simulink model "Motor_pos_ref"  (R2020b)
settings: Solver=ode45  StartTime=0.0  StopTime=0.2  RelTol=1e-3
values from neighbouring files (symbols this model uses):
  b = 3.5077E-6    [DataDictionary.sldd]
  J = 3.2284E-6    [DataDictionary.sldd]
  Ke = 0.0274    [DataDictionary.sldd]
  Kt = 0.0274    [DataDictionary.sldd]
  L = 2.75E-6    [DataDictionary.sldd]
  R = 4.0    [DataDictionary.sldd]
settings Model: DataDictionary=DataDictionary.sldd  PacingRate=1000000  Creator=abhin  LastModifiedBy=abhin
settings DataIOCC: SaveOutput=off  SaveTime=off

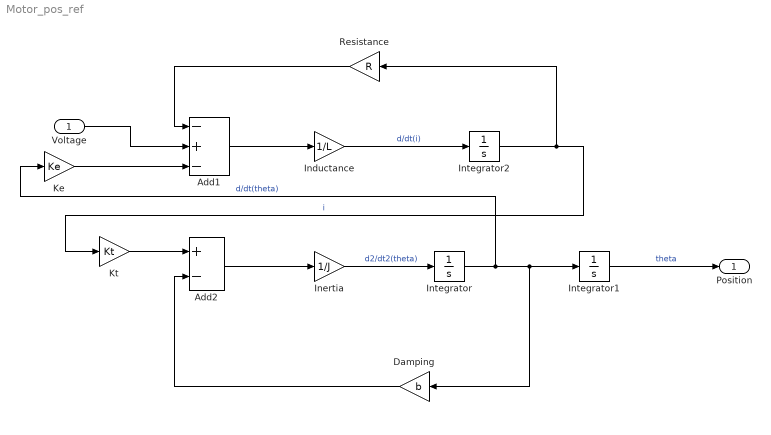
== system Motor_pos_ref ==
  Voltage : Inport  OutDataTypeStr=double  PortDimensions=1  SampleTime=0
  Add1 : Sum  Inputs=-+-
  Add2 : Sum  Inputs=+-
  Damping : Gain  Gain=b
  Inductance : Gain  Gain=1/L
  Inertia : Gain  Gain=1/J
  Integrator : Integrator
  Integrator1 : Integrator
  Integrator2 : Integrator
  Ke : Gain  Gain=Ke
  Kt : Gain  Gain=Kt
  Resistance : Gain  Gain=R
  Position : Outport  OutDataTypeStr=double  PortDimensions=1  SampleTime=0
  wires:
  Integrator1/1 -> Position/1  "theta"
  Inductance/1 -> Integrator2/1  "d/dt(i)"
  Integrator2/1 -> Kt/1, Resistance/1  "i"
  Resistance/1 -> Add1/1
  Integrator/1 -> Integrator1/1, Damping/1, Ke/1  "d/dt(theta)"
  Inertia/1 -> Integrator/1  "d2/dt2(theta)"
  Add2/1 -> Inertia/1
  Voltage/1 -> Add1/2
  Add1/1 -> Inductance/1
  Kt/1 -> Add2/1
  Damping/1 -> Add2/2
  Ke/1 -> Add1/3
